simulink model "Test01"  (Simulink 5.0)
settings: Solver=FixedStepDiscrete  StartTime=0.0  StopTime=inf  FixedStep=1/100000  RelTol=1e-3
settings Model: LastModifiedBy=Administrator  RTWOptions="-aEnforceIntegerDowncast=1 -aExtMode=0 -aExtModeTesting=0 -aFoldNonRolledExpr=1 -aForceParamTrailComments=0 -aGenerateComments=1 -aGenerateReport=0 -aIgnoreCustomStorageClasses=1 -aIncDataTypeInIds=0 -aIncHierarchyInIds=0 -aInlineInvariantSignals=1 -aInlineParameters=0 -aInlinedPrmAccess=\"Literals\" -aLocalBlockOutputs=1 -aLogVarNameModifier=\"rt_\" -aMaxRTWIdLen=31 -aPrefixModelToSubsysFcnNames=1 -aRTWVerbose=1 -aRollThreshold=5 -aShowEliminatedStatements=0"

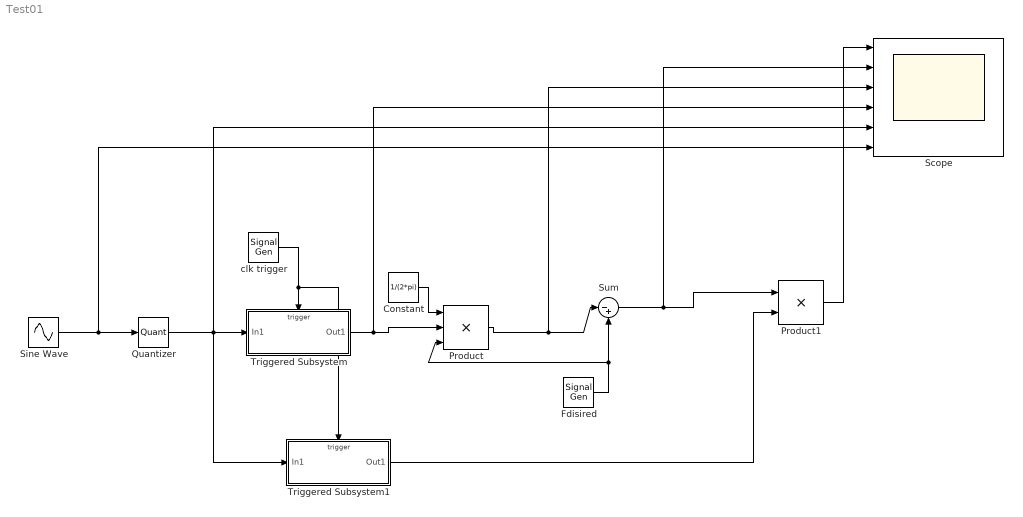
== system Test01 ==
  Constant : Constant  Value=1/(2*pi)
  Fdisired : SignalGenerator  WaveForm=square  Frequency=2000
  Product : Product  Inputs=3  SaturateOnIntegerOverflow=on
  Product1 : Product  SaturateOnIntegerOverflow=on
  Quantizer : Quantizer  QuantizationInterval=2/(2^3)
  Scope : Scope  NumInputPorts=6
      settings: TickLabels=on  TimeRange=0.0002459751434628343  YMin=-1~-1~-0.25~1.3~-0.75~-0.9  YMax=1~1~0.25~1.575~0.5~0.5
  Sine Wave : Sin  Frequency=2*pi*1000  SampleTime=0
  Sum : Sum  Inputs=|-+  SaturateOnIntegerOverflow=on
  Triggered Subsystem : Subsystem  TreatAsAtomicUnit=on
  Triggered Subsystem1 : Subsystem  TreatAsAtomicUnit=on
  clk trigger : SignalGenerator  WaveForm=square  Frequency=4500
  wires:
  Sine Wave/1 -> Quantizer/1, Scope/6
  Quantizer/1 -> Triggered Subsystem/1(In1), Scope/5, Triggered Subsystem1/1(In1)
  clk trigger/1 -> Triggered Subsystem/Trigger, Triggered Subsystem1/Trigger
  Product/1 -> Sum/1, Scope/3
  Sum/1 -> Product1/1, Scope/2
  Product1/1 -> Scope/1
  Triggered Subsystem/1(Out1) -> Product/2, Scope/4
  Triggered Subsystem1/1(Out1) -> Product1/2
  Constant/1 -> Product/1
  Fdisired/1 -> Sum/2, Product/3

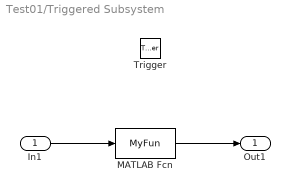
== system Test01/Triggered Subsystem ==
  In1 : Inport
  Trigger : TriggerPort
  MATLAB Fcn : MATLABFcn  MATLABFcn=MyFun
  Out1 : Outport
  wires:
  In1/1 -> MATLAB Fcn/1
  MATLAB Fcn/1 -> Out1/1

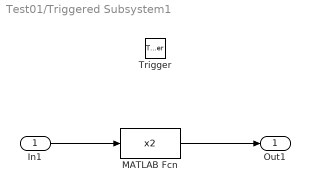
== system Test01/Triggered Subsystem1 ==
  In1 : Inport
  Trigger : TriggerPort
  MATLAB Fcn : MATLABFcn  MATLABFcn=x2
  Out1 : Outport
  wires:
  In1/1 -> MATLAB Fcn/1
  MATLAB Fcn/1 -> Out1/1
